simulink model "mrefrobotarm_modified_previous_y_previous_u_previous_ref_prepro"  (R2018b)
settings: Solver=FixedStepAuto  StartTime=0.0  StopTime=10  RelTol=1e-3  AbsTol=1e-6
undefined symbols (not defined in the file or in its folder): cc, options
libraries: neural x594, simulink x1
(part 20 of 22)

== system mrefrobotarm_modified_previous_y_previous_u_previous_ref_prepro/pre_0.001/Layer 3/Delays 1 ==
  "p{3}" : Inport  PortDimensions=30
      mask Display: e = 0.06;c1 = [120 230 180]/255;c2 = ([120 230 180]+0)/(256+128);c3 = ([120 230 180]+128)/(256+128);patch([0 1 1 0],[0 0 1 1],c1);patch([0 1 1 1-e 1-e 0+e],[0 0 1 1-e 0+e 0+e],c2);patch([0 0 1 1-e 0+e 0+e],[0 1 1 1-e 1-e 0+e],c3);plot([0 1 1 0 0],[0 0 1 1 0]);
  mux : Mux  Inputs=1
      mask Display: e = 0.06;c1 = [120 150 230]/255;c2 = ([120 150 230]+0)/383;c3 = ([120 150 230]+128)/383;patch([0 1 1 0],[0 0 1 1],c1);patch([0 1 1 1-e 1-e 0+e],[0 0 1 1-e 0+e 0+e],c2);patch([0 0 1 1-e 0+e 0+e],[0 1 1 1-e 1-e 0+e],c3);plot([0 1 1 0 0],[0 0 1 1 0]);disp('Mux')
  "pd{3,2}" : Outport
      mask Display: e = 0.06;c1 = [120 230 180]/255;c2 = ([120 230 180]+0)/(256+128);c3 = ([120 230 180]+128)/(256+128);patch([0 1 1 0],[0 0 1 1],c1);patch([0 1 1 1-e 1-e 0+e],[0 0 1 1-e 0+e 0+e],c2);patch([0 0 1 1-e 0+e 0+e],[0 1 1 1-e 1-e 0+e],c3);plot([0 1 1 0 0],[0 0 1 1 0]);
  wires:
  "p{3}"/1 -> mux/1
  mux/1 -> "pd{3,2}"/1

== system mrefrobotarm_modified_previous_y_previous_u_previous_ref_prepro/pre_0.001/Layer 3/LW{3,2} ==
  "ad{3,2}" : Inport  PortDimensions=30
      mask Display: e = 0.06;c1 = [120 230 180]/255;c2 = ([120 230 180]+0)/(256+128);c3 = ([120 230 180]+128)/(256+128);patch([0 1 1 0],[0 0 1 1],c1);patch([0 1 1 1-e 1-e 0+e],[0 0 1 1-e 0+e 0+e],c2);patch([0 0 1 1-e 0+e 0+e],[0 1 1 1-e 1-e 0+e],c3);plot([0 1 1 0 0],[0 0 1 1 0]);
  "IW{3,2}(1,:)'" : Constant  Value=[0.436114134671065689641267226761556230485439300537109375;0.4897108664989697768277210343512706458568572998046875;0.265158589575804126692304407697520218789577484130859375;-0.51659794668614644752580034037237055599689483642578125;0.5796996893935404404629707642016001045703887939453125;-0.57276838291900122879241052942234091460704803466796875;0.335826299327664390403924699057824909687042236328125;-0.261032698694444509346368477054056711494922637939453125;0.1045260610150008651064723608214990235865116119384765625;0.49111728847109958895345016571809537708759307861328125;-0.42848603195214407524105126867652870714664459228515625;-0.101925406868263734860846625451813451945781707763671875;-0.175991462046761026893904045209637843072414398193359375;-0.010501595203579773551982867729748249985277652740478515625;0.299745457740388243639273468943429179489612579345703125;-0.1603921728348352282456090733830933459103107452392578125;0.066959779095569327278525406654807738959789276123046875;-0.450890234310093951375364440536941401660442352294921875;-0.51157208381028629329279056037194095551967620849609375;-0.09288836924470354750038580959881073795258998870849609375;0.50675121237872833290794005733914673328399658203125;0.1206441884120259266932606578848208300769329071044921875;0.11866864954212101579411609009184758178889751434326171875;-0.0393519848847962150362178590512485243380069732666015625;-0.242185273598383654647392404513084329664707183837890625;-0.164235090509567693839443336401018314063549041748046875;0.33195926443744749878561606237781234085559844970703125;0.0119212193619771915364946579529714654199779033660888671875;-0.068550038750629205264175425327266566455364227294921875;-0.0692097648270704468576042245331336744129657745361328125]
      mask Display: e = 0.06;c1 = [120 150 230]/255;c2 = ([120 150 230]+0)/383;c3 = ([120 150 230]+128)/383;patch([0 1 1 0],[0 0 1 1],c1);patch([0 1 1 1-e 1-e 0+e],[0 0 1 1-e 0+e 0+e],c2);patch([0 0 1 1-e 0+e 0+e],[0 1 1 1-e 1-e 0+e],c3);plot([0 1 1 0 0],[0 0 1 1 0]);disp('weights');
  Mux : Mux  Inputs=1
      mask Display: e = 0.06;c1 = [120 150 230]/255;c2 = ([120 150 230]+0)/383;c3 = ([120 150 230]+128)/383;patch([0 1 1 0],[0 0 1 1],c1);patch([0 1 1 1-e 1-e 0+e],[0 0 1 1-e 0+e 0+e],c2);patch([0 0 1 1-e 0+e 0+e],[0 1 1 1-e 1-e 0+e],c3);plot([0 1 1 0 0],[0 0 1 1 0]);disp('Mux');
  dotprod1 : neural/Weight Functions/dotprod
  "lz{3,2}" : Outport
      mask Display: e = 0.06;c1 = [120 230 180]/255;c2 = ([120 230 180]+0)/(256+128);c3 = ([120 230 180]+128)/(256+128);patch([0 1 1 0],[0 0 1 1],c1);patch([0 1 1 1-e 1-e 0+e],[0 0 1 1-e 0+e 0+e],c2);patch([0 0 1 1-e 0+e 0+e],[0 1 1 1-e 1-e 0+e],c3);plot([0 1 1 0 0],[0 0 1 1 0]);
  wires:
  "IW{3,2}(1,:)'"/1 -> dotprod1/1
  "ad{3,2}"/1 -> dotprod1/2
  dotprod1/1 -> Mux/1
  Mux/1 -> "lz{3,2}"/1

== system mrefrobotarm_modified_previous_y_previous_u_previous_ref_prepro/pre_0.01/Layer 1/Delays 1 ==
  "p{1}" : Inport  PortDimensions=10
      mask Display: e = 0.06;c1 = [120 230 180]/255;c2 = ([120 230 180]+0)/(256+128);c3 = ([120 230 180]+128)/(256+128);patch([0 1 1 0],[0 0 1 1],c1);patch([0 1 1 1-e 1-e 0+e],[0 0 1 1-e 0+e 0+e],c2);patch([0 0 1 1-e 0+e 0+e],[0 1 1 1-e 1-e 0+e],c3);plot([0 1 1 0 0],[0 0 1 1 0]);
  mux : Mux  Inputs=1
      mask Display: e = 0.06;c1 = [120 150 230]/255;c2 = ([120 150 230]+0)/383;c3 = ([120 150 230]+128)/383;patch([0 1 1 0],[0 0 1 1],c1);patch([0 1 1 1-e 1-e 0+e],[0 0 1 1-e 0+e 0+e],c2);patch([0 0 1 1-e 0+e 0+e],[0 1 1 1-e 1-e 0+e],c3);plot([0 1 1 0 0],[0 0 1 1 0]);disp('Mux')
  "pd{1,1}" : Outport
      mask Display: e = 0.06;c1 = [120 230 180]/255;c2 = ([120 230 180]+0)/(256+128);c3 = ([120 230 180]+128)/(256+128);patch([0 1 1 0],[0 0 1 1],c1);patch([0 1 1 1-e 1-e 0+e],[0 0 1 1-e 0+e 0+e],c2);patch([0 0 1 1-e 0+e 0+e],[0 1 1 1-e 1-e 0+e],c3);plot([0 1 1 0 0],[0 0 1 1 0]);
  wires:
  "p{1}"/1 -> mux/1
  mux/1 -> "pd{1,1}"/1

== system mrefrobotarm_modified_previous_y_previous_u_previous_ref_prepro/pre_0.01/Layer 1/IW{1,1} ==
  "pd{1,1}" : Inport  PortDimensions=10
      mask Display: e = 0.06;c1 = [120 230 180]/255;c2 = ([120 230 180]+0)/(256+128);c3 = ([120 230 180]+128)/(256+128);patch([0 1 1 0],[0 0 1 1],c1);patch([0 1 1 1-e 1-e 0+e],[0 0 1 1-e 0+e 0+e],c2);patch([0 0 1 1-e 0+e 0+e],[0 1 1 1-e 1-e 0+e],c3);plot([0 1 1 0 0],[0 0 1 1 0]);
  "IW{1,1}(1,:)'" : Constant  Value=[-5.85624074115564940967715301667340099811553955078125;3.51680446128212498280163345043547451496124267578125;0.6347381482262941521099719466292299330234527587890625;1.7803816056595789252270378710818476974964141845703125;-1.2333050429232244038502130933920852839946746826171875;-0.1301107597361087775400534383152262307703495025634765625;3.545860369137638468117756929132156074047088623046875;-2.8459252595942228225567305344156920909881591796875;-0.3393944679271430064915193725028075277805328369140625;0.332423639089425126957877409950015135109424591064453125]
      mask Display: e = 0.06;c1 = [120 150 230]/255;c2 = ([120 150 230]+0)/383;c3 = ([120 150 230]+128)/383;patch([0 1 1 0],[0 0 1 1],c1);patch([0 1 1 1-e 1-e 0+e],[0 0 1 1-e 0+e 0+e],c2);patch([0 0 1 1-e 0+e 0+e],[0 1 1 1-e 1-e 0+e],c3);plot([0 1 1 0 0],[0 0 1 1 0]);disp('Weights');
  "IW{1,1}(10,:)'" : Constant  Value=[5.5438114168611445364831524784676730632781982421875;-2.074847987877894706088000020827166736125946044921875;-1.92727949100788986669385849381797015666961669921875;-0.467908740727801586434253522384096868336200714111328125;-2.076676504568512715565020698704756796360015869140625;-0.10576368682021698719442071023877360858023166656494140625;5.00949759583771214721537035075016319751739501953125;-3.03922330836093834705025074072182178497314453125;0.604367742739750468672355054877698421478271484375;-3.819841634701873100965485718916170299053192138671875]
      mask Display: e = 0.06;c1 = [120 150 230]/255;c2 = ([120 150 230]+0)/383;c3 = ([120 150 230]+128)/383;patch([0 1 1 0],[0 0 1 1],c1);patch([0 1 1 1-e 1-e 0+e],[0 0 1 1-e 0+e 0+e],c2);patch([0 0 1 1-e 0+e 0+e],[0 1 1 1-e 1-e 0+e],c3);plot([0 1 1 0 0],[0 0 1 1 0]);disp('Weights');
  "IW{1,1}(11,:)'" : Constant  Value=[1.801450365151530785823297264869324862957000732421875;2.5403773096062547409701437572948634624481201171875;-0.61133654619760935400307744203018955886363983154296875;0.2245239888465724031885173417322221212089061737060546875;-4.25834432503798243629944408894516527652740478515625;-0.456781073421577143989225078257732093334197998046875;1.90877776482296379612080272636376321315765380859375;-0.2448749812280913429329842756487778387963771820068359375;2.974360199360491119335847542970441281795501708984375;0.752977482462759528658580165938474237918853759765625]
      mask Display: e = 0.06;c1 = [120 150 230]/255;c2 = ([120 150 230]+0)/383;c3 = ([120 150 230]+128)/383;patch([0 1 1 0],[0 0 1 1],c1);patch([0 1 1 1-e 1-e 0+e],[0 0 1 1-e 0+e 0+e],c2);patch([0 0 1 1-e 0+e 0+e],[0 1 1 1-e 1-e 0+e],c3);plot([0 1 1 0 0],[0 0 1 1 0]);disp('Weights');
  "IW{1,1}(12,:)'" : Constant  Value=[-5.88547165882157674587915607844479382038116455078125;0.3690016789117473994252804914140142500400543212890625;5.43454272118004677594171880627982318401336669921875;2.021324955409448786980419754399918019771575927734375;3.118231972581463562477210871293209493160247802734375;-4.67881290747909162064388510771095752716064453125;-1.560839517955373789703799047856591641902923583984375;1.316600991380263874219735953374765813350677490234375;-2.9123006538206706039773052907548844814300537109375;-0.36660783874813229754607846189173869788646697998046875]
      mask Display: e = 0.06;c1 = [120 150 230]/255;c2 = ([120 150 230]+0)/383;c3 = ([120 150 230]+128)/383;patch([0 1 1 0],[0 0 1 1],c1);patch([0 1 1 1-e 1-e 0+e],[0 0 1 1-e 0+e 0+e],c2);patch([0 0 1 1-e 0+e 0+e],[0 1 1 1-e 1-e 0+e],c3);plot([0 1 1 0 0],[0 0 1 1 0]);disp('Weights');
  "IW{1,1}(13,:)'" : Constant  Value=[4.4862364253392978952206249232403934001922607421875;-2.21359337096940311795378875103779137134552001953125;-3.6510555857054516337711902451701462268829345703125;-0.59044303803139985831194280763156712055206298828125;4.35225243695406671662340158945880830287933349609375;-0.944076425101286087482321818242780864238739013671875;0.601137947571718456174494349397718906402587890625;-0.9102507336520961889192449234542436897754669189453125;-2.040783866186438810785830355598591268062591552734375;1.14248211452239889496240721200592815876007080078125]
      mask Display: e = 0.06;c1 = [120 150 230]/255;c2 = ([120 150 230]+0)/383;c3 = ([120 150 230]+128)/383;patch([0 1 1 0],[0 0 1 1],c1);patch([0 1 1 1-e 1-e 0+e],[0 0 1 1-e 0+e 0+e],c2);patch([0 0 1 1-e 0+e 0+e],[0 1 1 1-e 1-e 0+e],c3);plot([0 1 1 0 0],[0 0 1 1 0]);disp('Weights');
  "IW{1,1}(14,:)'" : Constant  Value=[2.96005758962551634994042615289799869060516357421875;-2.628426232952859376013066139421425759792327880859375;0.9426964090625158387837245754781179130077362060546875;-2.009528625793982836711393247242085635662078857421875;4.98013932269017356446738631348125636577606201171875;-2.84339358174093081998989873682148754596710205078125;-1.499753220486744975659121337230317294597625732421875;0.61186224711551628896444299243739806115627288818359375;-0.91867019710147157507407200682791881263256072998046875;-1.1056470699375766653105301884352229535579681396484375]
      mask Display: e = 0.06;c1 = [120 150 230]/255;c2 = ([120 150 230]+0)/383;c3 = ([120 150 230]+128)/383;patch([0 1 1 0],[0 0 1 1],c1);patch([0 1 1 1-e 1-e 0+e],[0 0 1 1-e 0+e 0+e],c2);patch([0 0 1 1-e 0+e 0+e],[0 1 1 1-e 1-e 0+e],c3);plot([0 1 1 0 0],[0 0 1 1 0]);disp('Weights');
  "IW{1,1}(15,:)'" : Constant  Value=[1.3405973719274850708416124689392745494842529296875;-0.94740730540068518461538360497797839343547821044921875;-0.8051968085434351163343080770573578774929046630859375;0.8401875525177968651036053415737114846706390380859375;-2.38333203591385522912560190889053046703338623046875;2.247255001731979451307097406242974102497100830078125;-2.1907243293222418145660412847064435482025146484375;1.393962444028848945976051254547201097011566162109375;-2.9782811404097788710032546077854931354522705078125;-3.071191113830036290011094024521298706531524658203125]
      mask Display: e = 0.06;c1 = [120 150 230]/255;c2 = ([120 150 230]+0)/383;c3 = ([120 150 230]+128)/383;patch([0 1 1 0],[0 0 1 1],c1);patch([0 1 1 1-e 1-e 0+e],[0 0 1 1-e 0+e 0+e],c2);patch([0 0 1 1-e 0+e 0+e],[0 1 1 1-e 1-e 0+e],c3);plot([0 1 1 0 0],[0 0 1 1 0]);disp('Weights');
  "IW{1,1}(16,:)'" : Constant  Value=[5.24956005510203294051052580471150577068328857421875;-3.123270889222998558665267410106025636196136474609375;-2.899628478866194125629363043117336928844451904296875;1.2721033387022446792258278946974314749240875244140625;-6.7373528318352189359075055108405649662017822265625;4.95546573290953151769144824356772005558013916015625;0.53229393194607588224442906721378676593303680419921875;1.3107157379762164328695916992728598415851593017578125;-6.4141498126504306043216274701990187168121337890625;-1.688800676216443807931000264943577349185943603515625]
      mask Display: e = 0.06;c1 = [120 150 230]/255;c2 = ([120 150 230]+0)/383;c3 = ([120 150 230]+128)/383;patch([0 1 1 0],[0 0 1 1],c1);patch([0 1 1 1-e 1-e 0+e],[0 0 1 1-e 0+e 0+e],c2);patch([0 0 1 1-e 0+e 0+e],[0 1 1 1-e 1-e 0+e],c3);plot([0 1 1 0 0],[0 0 1 1 0]);disp('Weights');
  "IW{1,1}(17,:)'" : Constant  Value=[0.402854375334637915262447904751752503216266632080078125;-1.9260767289406282021246852309559471905231475830078125;0.78951047299180476812807683018036186695098876953125;0.68164611125391871837564394809305667877197265625;-0.634424106110297092442351640784181654453277587890625;0.1365768899834514382707340018896502442657947540283203125;1.9467877645893822968758968272595666348934173583984375;-0.913545588347322468081301849451847374439239501953125;1.6488021045101197703530715443775989115238189697265625;-0.22812449883821361851232722983695566654205322265625]
      mask Display: e = 0.06;c1 = [120 150 230]/255;c2 = ([120 150 230]+0)/383;c3 = ([120 150 230]+128)/383;patch([0 1 1 0],[0 0 1 1],c1);patch([0 1 1 1-e 1-e 0+e],[0 0 1 1-e 0+e 0+e],c2);patch([0 0 1 1-e 0+e 0+e],[0 1 1 1-e 1-e 0+e],c3);plot([0 1 1 0 0],[0 0 1 1 0]);disp('Weights');
  "IW{1,1}(18,:)'" : Constant  Value=[-3.926344015276355126076168744475580751895904541015625;2.64736178851262682343303822563029825687408447265625;1.4944123035889393946717973449267446994781494140625;-1.548625935119756658053802311769686639308929443359375;2.158669751416033566471242011175490915775299072265625;-0.3860689796058196510131210743566043674945831298828125;-1.255149649516599463794364055502228438854217529296875;0.5499562614605004728929316115682013332843780517578125;1.4076190893442135365631884269532747566699981689453125;-1.68961743441577372237816234701313078403472900390625]
      mask Display: e = 0.06;c1 = [120 150 230]/255;c2 = ([120 150 230]+0)/383;c3 = ([120 150 230]+128)/383;patch([0 1 1 0],[0 0 1 1],c1);patch([0 1 1 1-e 1-e 0+e],[0 0 1 1-e 0+e 0+e],c2);patch([0 0 1 1-e 0+e 0+e],[0 1 1 1-e 1-e 0+e],c3);plot([0 1 1 0 0],[0 0 1 1 0]);disp('Weights');
  "IW{1,1}(19,:)'" : Constant  Value=[-8.6575548675962945566197959124110639095306396484375;4.10379744179784466950877686031162738800048828125;-0.327724649637724685380391065336880274116992950439453125;3.97567807798125461005156466853804886341094970703125;3.70194788223165627272237543365918099880218505859375;-1.2007687177355277352575058102956973016262054443359375;-2.094451910380683568035919961403124034404754638671875;0.6931746778662428720707566753844730556011199951171875;0.390829399024751278357570072330418042838573455810546875;3.424383189735958676891414143028669059276580810546875]
      mask Display: e = 0.06;c1 = [120 150 230]/255;c2 = ([120 150 230]+0)/383;c3 = ([120 150 230]+128)/383;patch([0 1 1 0],[0 0 1 1],c1);patch([0 1 1 1-e 1-e 0+e],[0 0 1 1-e 0+e 0+e],c2);patch([0 0 1 1-e 0+e 0+e],[0 1 1 1-e 1-e 0+e],c3);plot([0 1 1 0 0],[0 0 1 1 0]);disp('Weights');
  "IW{1,1}(2,:)'" : Constant  Value=[2.6125118629305763562342690420337021350860595703125;-1.37514288325557654246722449897788465023040771484375;-1.401681826106581763013991803745739161968231201171875;0.83219132133275397489313718324410729110240936279296875;-1.953893972122157318693780325702391564846038818359375;0.69612144520550833792782441378221847116947174072265625;1.7696692580941599803878716556937433779239654541015625;-1.5785633815546535885232515283860266208648681640625;-3.442944793421773841402000471134670078754425048828125;0.68140069773722711232721849228255450725555419921875]
      mask Display: e = 0.06;c1 = [120 150 230]/255;c2 = ([120 150 230]+0)/383;c3 = ([120 150 230]+128)/383;patch([0 1 1 0],[0 0 1 1],c1);patch([0 1 1 1-e 1-e 0+e],[0 0 1 1-e 0+e 0+e],c2);patch([0 0 1 1-e 0+e 0+e],[0 1 1 1-e 1-e 0+e],c3);plot([0 1 1 0 0],[0 0 1 1 0]);disp('Weights');
  "IW{1,1}(20,:)'" : Constant  Value=[-5.82456522810500754161466829827986657619476318359375;4.77771073300586035514925242750905454158782958984375;2.22666821103919065905074603506363928318023681640625;-2.07154279514932770922541749314405024051666259765625;1.984621844522302058777540878509171307086944580078125;0.81260359941105109182757360031246207654476165771484375;-1.7979220800818911385476894793100655078887939453125;-0.19148413309093204048849656828679144382476806640625;3.266091133828860737509103273623622953891754150390625;-0.423175203307374736549917315642233006656169891357421875]
      mask Display: e = 0.06;c1 = [120 150 230]/255;c2 = ([120 150 230]+0)/383;c3 = ([120 150 230]+128)/383;patch([0 1 1 0],[0 0 1 1],c1);patch([0 1 1 1-e 1-e 0+e],[0 0 1 1-e 0+e 0+e],c2);patch([0 0 1 1-e 0+e 0+e],[0 1 1 1-e 1-e 0+e],c3);plot([0 1 1 0 0],[0 0 1 1 0]);disp('Weights');
  "IW{1,1}(21,:)'" : Constant  Value=[-2.6788162832066291230148635804653167724609375;1.531265910973661714677973577636294066905975341796875;-1.2272697973190014320010732262744568288326263427734375;0.2462738275440067570176694289330043829977512359619140625;3.7563299795286670956784291774965822696685791015625;-2.676750026289990369576798912021331489086151123046875;2.749977990810542838318042413447983562946319580078125;-2.43343537079067306905244549852795898914337158203125;-3.120985268643997390114463996724225580692291259765625;1.3113749338071869487976073287427425384521484375]
      mask Display: e = 0.06;c1 = [120 150 230]/255;c2 = ([120 150 230]+0)/383;c3 = ([120 150 230]+128)/383;patch([0 1 1 0],[0 0 1 1],c1);patch([0 1 1 1-e 1-e 0+e],[0 0 1 1-e 0+e 0+e],c2);patch([0 0 1 1-e 0+e 0+e],[0 1 1 1-e 1-e 0+e],c3);plot([0 1 1 0 0],[0 0 1 1 0]);disp('Weights');
  "IW{1,1}(22,:)'" : Constant  Value=[-2.331678787855488987901253494783304631710052490234375;1.9175273555104686007410919046378694474697113037109375;2.785754327334096114299200053210370242595672607421875;1.220232959880296785826203631586395204067230224609375;3.930124642441815918658676309860311448574066162109375;-0.9763831564017639852437469016877003014087677001953125;-0.5288300752090524525783621356822550296783447265625;-0.53467152456522060166577148265787400305271148681640625;3.027168159407801706350937820388935506343841552734375;-2.546789484386377200308970714104361832141876220703125]
      mask Display: e = 0.06;c1 = [120 150 230]/255;c2 = ([120 150 230]+0)/383;c3 = ([120 150 230]+128)/383;patch([0 1 1 0],[0 0 1 1],c1);patch([0 1 1 1-e 1-e 0+e],[0 0 1 1-e 0+e 0+e],c2);patch([0 0 1 1-e 0+e 0+e],[0 1 1 1-e 1-e 0+e],c3);plot([0 1 1 0 0],[0 0 1 1 0]);disp('Weights');
  "IW{1,1}(23,:)'" : Constant  Value=[-3.297749992552132969336753376410342752933502197265625;0.95345391607309759596233789125108160078525543212890625;1.3085273842947042766127196955494582653045654296875;-2.09606923060831373817336498177610337734222412109375;0.6649085374571017670319861281313933432102203369140625;-2.605191632574497706542615560465492308139801025390625;-0.2086664202659928302185932125212275423109531402587890625;0.29301975068497665422029285764438100159168243408203125;0.0533424003255774381582199339391081593930721282958984375;-0.9746507344559234287117988060344941914081573486328125]
      mask Display: e = 0.06;c1 = [120 150 230]/255;c2 = ([120 150 230]+0)/383;c3 = ([120 150 230]+128)/383;patch([0 1 1 0],[0 0 1 1],c1);patch([0 1 1 1-e 1-e 0+e],[0 0 1 1-e 0+e 0+e],c2);patch([0 0 1 1-e 0+e 0+e],[0 1 1 1-e 1-e 0+e],c3);plot([0 1 1 0 0],[0 0 1 1 0]);disp('Weights');
  "IW{1,1}(24,:)'" : Constant  Value=[5.26403541711713796047433788771741092205047607421875;-4.350305274247940445775384432636201381683349609375;-2.446240935645905612005890361615456640720367431640625;0.281055804546570364710333933544461615383625030517578125;1.50024635213031043434739331132732331752777099609375;-4.03994831318534775022044414072297513484954833984375;-1.835789247584131533841400596429593861103057861328125;1.1544983756443236710964583835448138415813446044921875;1.348684999744826473744296890799887478351593017578125;-2.47782798748131316557419268065132200717926025390625]
      mask Display: e = 0.06;c1 = [120 150 230]/255;c2 = ([120 150 230]+0)/383;c3 = ([120 150 230]+128)/383;patch([0 1 1 0],[0 0 1 1],c1);patch([0 1 1 1-e 1-e 0+e],[0 0 1 1-e 0+e 0+e],c2);patch([0 0 1 1-e 0+e 0+e],[0 1 1 1-e 1-e 0+e],c3);plot([0 1 1 0 0],[0 0 1 1 0]);disp('Weights');
  "IW{1,1}(25,:)'" : Constant  Value=[-3.7163175636467347118241377756930887699127197265625;0.52039148612197172472093598116771318018436431884765625;0.62464525370229118106379928576643578708171844482421875;1.1292601515886386831510890260688029229640960693359375;4.03204641347660075467729257070459425449371337890625;-3.35339086600971025831086080870591104030609130859375;-0.67736203672771699846322235316620208323001861572265625;1.1033568521567953535367223594221286475658416748046875;2.1720579810827533862038762890733778476715087890625;0.294348933198287754375854774480103515088558197021484375]
      mask Display: e = 0.06;c1 = [120 150 230]/255;c2 = ([120 150 230]+0)/383;c3 = ([120 150 230]+128)/383;patch([0 1 1 0],[0 0 1 1],c1);patch([0 1 1 1-e 1-e 0+e],[0 0 1 1-e 0+e 0+e],c2);patch([0 0 1 1-e 0+e 0+e],[0 1 1 1-e 1-e 0+e],c3);plot([0 1 1 0 0],[0 0 1 1 0]);disp('Weights');
  "IW{1,1}(26,:)'" : Constant  Value=[7.68110421554345013106512851663865149021148681640625;-5.5806375133580292668966649216599762439727783203125;0.6474186917384816553067139466293156147003173828125;-0.25813591302558880347106651242938823997974395751953125;-7.25354088639611660482842125929892063140869140625;2.34772948867883091139674434089101850986480712890625;2.008143539473588479182808441692031919956207275390625;0.328548453086462022287861373115447349846363067626953125;0.66391334420801617621776813393807969987392425537109375;-1.7681702103446050866608629803522489964962005615234375]
      mask Display: e = 0.06;c1 = [120 150 230]/255;c2 = ([120 150 230]+0)/383;c3 = ([120 150 230]+128)/383;patch([0 1 1 0],[0 0 1 1],c1);patch([0 1 1 1-e 1-e 0+e],[0 0 1 1-e 0+e 0+e],c2);patch([0 0 1 1-e 0+e 0+e],[0 1 1 1-e 1-e 0+e],c3);plot([0 1 1 0 0],[0 0 1 1 0]);disp('Weights');
  "IW{1,1}(27,:)'" : Constant  Value=[-3.88890360968008419462194069637916982173919677734375;1.807719452135531756908903844305314123630523681640625;1.8443906482025564930182781608891673386096954345703125;0.05960729976508481742225598054574220441281795501708984375;6.41662600072029309927756912657059729099273681640625;-4.731342225276449653392774052917957305908203125;-1.9683220855801606408164161621243692934513092041015625;-0.155691989537033170787339031448937021195888519287109375;1.5052831323353388359720383959938772022724151611328125;3.0499443373096735143690239056013524532318115234375]
      mask Display: e = 0.06;c1 = [120 150 230]/255;c2 = ([120 150 230]+0)/383;c3 = ([120 150 230]+128)/383;patch([0 1 1 0],[0 0 1 1],c1);patch([0 1 1 1-e 1-e 0+e],[0 0 1 1-e 0+e 0+e],c2);patch([0 0 1 1-e 0+e 0+e],[0 1 1 1-e 1-e 0+e],c3);plot([0 1 1 0 0],[0 0 1 1 0]);disp('Weights');
  "IW{1,1}(28,:)'" : Constant  Value=[-2.08873314887912808757164384587667882442474365234375;-2.177558277080478443821220935205928981304168701171875;1.85911414065590374633529791026376187801361083984375;0.7786322163372434435046898215659894049167633056640625;-2.878435651152690955001389738754369318485260009765625;0.85485495305713066205299810462747700512409210205078125;-0.544214717952030024861187484930269420146942138671875;1.2201975643732592136103676239144988358020782470703125;1.9343350066125617470191855318262241780757904052734375;-0.1590528401144102321751461204257793724536895751953125]
      mask Display: e = 0.06;c1 = [120 150 230]/255;c2 = ([120 150 230]+0)/383;c3 = ([120 150 230]+128)/383;patch([0 1 1 0],[0 0 1 1],c1);patch([0 1 1 1-e 1-e 0+e],[0 0 1 1-e 0+e 0+e],c2);patch([0 0 1 1-e 0+e 0+e],[0 1 1 1-e 1-e 0+e],c3);plot([0 1 1 0 0],[0 0 1 1 0]);disp('Weights');
  "IW{1,1}(29,:)'" : Constant  Value=[-3.3140155268266173749225345090962946414947509765625;2.22866180250222978287411024211905896663665771484375;-0.20167459266773357651203468776657246053218841552734375;-0.1575369015674890904588067996883182786405086517333984375;-3.381821830384472260533357257372699677944183349609375;1.2952284826152082874983761939802207052707672119140625;-1.1796565663488285391480303587741218507289886474609375;3.439748069590938595041507142013870179653167724609375;-3.675285077898163610399251410854049026966094970703125;-2.262756383297438222967912224703468382358551025390625]
      mask Display: e = 0.06;c1 = [120 150 230]/255;c2 = ([120 150 230]+0)/383;c3 = ([120 150 230]+128)/383;patch([0 1 1 0],[0 0 1 1],c1);patch([0 1 1 1-e 1-e 0+e],[0 0 1 1-e 0+e 0+e],c2);patch([0 0 1 1-e 0+e 0+e],[0 1 1 1-e 1-e 0+e],c3);plot([0 1 1 0 0],[0 0 1 1 0]);disp('Weights');
  "IW{1,1}(3,:)'" : Constant  Value=[-0.56675888134729401901523715423536486923694610595703125;-0.34119466903833195470241435032221488654613494873046875;-0.39663512936999711921970401817816309630870819091796875;0.478829072563840885123909174581058323383331298828125;-3.366711754555829383406262422795407474040985107421875;3.2339992215156403432274601073004305362701416015625;-1.1517120277756067725505317866918630897998809814453125;1.4794355264062897248322769883088767528533935546875;-4.24056030156204588621449147467501461505889892578125;1.210775540611519485167946186265908181667327880859375]
      mask Display: e = 0.06;c1 = [120 150 230]/255;c2 = ([120 150 230]+0)/383;c3 = ([120 150 230]+128)/383;patch([0 1 1 0],[0 0 1 1],c1);patch([0 1 1 1-e 1-e 0+e],[0 0 1 1-e 0+e 0+e],c2);patch([0 0 1 1-e 0+e 0+e],[0 1 1 1-e 1-e 0+e],c3);plot([0 1 1 0 0],[0 0 1 1 0]);disp('Weights');
  "IW{1,1}(30,:)'" : Constant  Value=[-1.2533905500174207237051859920029528439044952392578125;-1.0861989916824443813681000392534770071506500244140625;1.396198612017170770371876642457209527492523193359375;2.860837090867893284240608409163542091846466064453125;-2.472957936277264234803396902862004935741424560546875;1.3823525587225502508914587451727129518985748291015625;-1.142285625577001528796472484827972948551177978515625;0.9551498948774297392816379215219058096408843994140625;1.1108403503011061719263352642883546650409698486328125;2.648168806111362183486335197812877595424652099609375]
      mask Display: e = 0.06;c1 = [120 150 230]/255;c2 = ([120 150 230]+0)/383;c3 = ([120 150 230]+128)/383;patch([0 1 1 0],[0 0 1 1],c1);patch([0 1 1 1-e 1-e 0+e],[0 0 1 1-e 0+e 0+e],c2);patch([0 0 1 1-e 0+e 0+e],[0 1 1 1-e 1-e 0+e],c3);plot([0 1 1 0 0],[0 0 1 1 0]);disp('Weights');
  "IW{1,1}(4,:)'" : Constant  Value=[-6.5853133771012029029634504695422947406768798828125;2.76263961904087285148534647305496037006378173828125;0.30869851091883881988309212829335592687129974365234375;0.4193313033892469565699911981937475502490997314453125;2.316828555632335362446383442147634923458099365234375;-1.1864510017739362535138525345246307551860809326171875;-0.485024537478817074909187567754997871816158294677734375;0.461871944816222346208434146319632418453693389892578125;0.433714380881770000808472786957281641662120819091796875;-3.204995011492357104287975744227878749370574951171875]
      mask Display: e = 0.06;c1 = [120 150 230]/255;c2 = ([120 150 230]+0)/383;c3 = ([120 150 230]+128)/383;patch([0 1 1 0],[0 0 1 1],c1);patch([0 1 1 1-e 1-e 0+e],[0 0 1 1-e 0+e 0+e],c2);patch([0 0 1 1-e 0+e 0+e],[0 1 1 1-e 1-e 0+e],c3);plot([0 1 1 0 0],[0 0 1 1 0]);disp('Weights');
  "IW{1,1}(5,:)'" : Constant  Value=[5.73852534707076689102223099325783550739288330078125;0.05805293153485781287859168742215842939913272857666015625;-3.04412521841268546296532804262824356555938720703125;-0.503981225017013922951036875019781291484832763671875;-2.549002892817883836329428959288634359836578369140625;3.2228411095297833099948547896929085254669189453125;0.97345814077867931501941711758263409137725830078125;-3.787924656487893226852747829980216920375823974609375;-0.60928514859972071615601407756912522017955780029296875;2.183424672023919210772646692930720746517181396484375]
      mask Display: e = 0.06;c1 = [120 150 230]/255;c2 = ([120 150 230]+0)/383;c3 = ([120 150 230]+128)/383;patch([0 1 1 0],[0 0 1 1],c1);patch([0 1 1 1-e 1-e 0+e],[0 0 1 1-e 0+e 0+e],c2);patch([0 0 1 1-e 0+e 0+e],[0 1 1 1-e 1-e 0+e],c3);plot([0 1 1 0 0],[0 0 1 1 0]);disp('Weights');
  "IW{1,1}(6,:)'" : Constant  Value=[-2.217512967826573255791799965663813054561614990234375;-0.58904066927541298692716509322053752839565277099609375;-2.49048429040009455803783566807396709918975830078125;-2.4578114385713103473563023726455867290496826171875;3.312526560791344110157297109253704547882080078125;1.2083392816733609098633905887254513800144195556640625;1.602648226646122164851249181083403527736663818359375;-0.067456206185177391976282024188549257814884185791015625;-1.8774466036302548399561374026234261691570281982421875;0.94688616102039180333349577267654240131378173828125]
      mask Display: e = 0.06;c1 = [120 150 230]/255;c2 = ([120 150 230]+0)/383;c3 = ([120 150 230]+128)/383;patch([0 1 1 0],[0 0 1 1],c1);patch([0 1 1 1-e 1-e 0+e],[0 0 1 1-e 0+e 0+e],c2);patch([0 0 1 1-e 0+e 0+e],[0 1 1 1-e 1-e 0+e],c3);plot([0 1 1 0 0],[0 0 1 1 0]);disp('Weights');
  "IW{1,1}(7,:)'" : Constant  Value=[-1.089049180437282604572146738064475357532501220703125;1.255433125095382518310316299903206527233123779296875;2.4781431225701648912718155770562589168548583984375;-1.0194681182791718310198803010280244052410125732421875;2.630481406433080149298575634020380675792694091796875;0.320844367893274695635597026921459473669528961181640625;2.25318642433378268918886533356271684169769287109375;0.475399692536651985452778035323717631399631500244140625;-2.68939142291155430797289227484725415706634521484375;-2.788639261698481863760434862342663109302520751953125]
      mask Display: e = 0.06;c1 = [120 150 230]/255;c2 = ([120 150 230]+0)/383;c3 = ([120 150 230]+128)/383;patch([0 1 1 0],[0 0 1 1],c1);patch([0 1 1 1-e 1-e 0+e],[0 0 1 1-e 0+e 0+e],c2);patch([0 0 1 1-e 0+e 0+e],[0 1 1 1-e 1-e 0+e],c3);plot([0 1 1 0 0],[0 0 1 1 0]);disp('Weights');
  "IW{1,1}(8,:)'" : Constant  Value=[2.392262476918522562385760465986095368862152099609375;0.177484958916592716615667768564890138804912567138671875;-1.7835335264594878168509239912964403629302978515625;0.0140831422173770814953996932672453112900257110595703125;2.43462897912698306157608385547064244747161865234375;0.29665149320045369751852604167652316391468048095703125;0.399042029318930235870510614404338411986827850341796875;-3.16678935948543571754498771042563021183013916015625;2.0553687128479456447394113638438284397125244140625;0.1463976569483515788316907446642289869487285614013671875]
      mask Display: e = 0.06;c1 = [120 150 230]/255;c2 = ([120 150 230]+0)/383;c3 = ([120 150 230]+128)/383;patch([0 1 1 0],[0 0 1 1],c1);patch([0 1 1 1-e 1-e 0+e],[0 0 1 1-e 0+e 0+e],c2);patch([0 0 1 1-e 0+e 0+e],[0 1 1 1-e 1-e 0+e],c3);plot([0 1 1 0 0],[0 0 1 1 0]);disp('Weights');
  "IW{1,1}(9,:)'" : Constant  Value=[5.0927416790097854715213543386198580265045166015625;-0.50360252949831874058617131595383398234844207763671875;-1.906654036515735839429908082820475101470947265625;-1.400523239361530780655584749183617532253265380859375;2.73113887691750534258972038514912128448486328125;-5.388534158780228011664803489111363887786865234375;1.99641404741776540276987361721694469451904296875;0.1001455352311608759663386081228964030742645263671875;-0.427650648383573306343663489315076731145381927490234375;-1.7623339402115936191961509393877349793910980224609375]
      mask Display: e = 0.06;c1 = [120 150 230]/255;c2 = ([120 150 230]+0)/383;c3 = ([120 150 230]+128)/383;patch([0 1 1 0],[0 0 1 1],c1);patch([0 1 1 1-e 1-e 0+e],[0 0 1 1-e 0+e 0+e],c2);patch([0 0 1 1-e 0+e 0+e],[0 1 1 1-e 1-e 0+e],c3);plot([0 1 1 0 0],[0 0 1 1 0]);disp('Weights');
  Mux : Mux  Inputs=30
      mask Display: e = 0.06;c1 = [120 150 230]/255;c2 = ([120 150 230]+0)/383;c3 = ([120 150 230]+128)/383;patch([0 1 1 0],[0 0 1 1],c1);patch([0 1 1 1-e 1-e 0+e],[0 0 1 1-e 0+e 0+e],c2);patch([0 0 1 1-e 0+e 0+e],[0 1 1 1-e 1-e 0+e],c3);plot([0 1 1 0 0],[0 0 1 1 0]);disp('Mux');
  dotprod{1..30} (30 alike) : neural/Weight Functions/dotprod
  "iz{1,1}" : Outport
      mask Display: e = 0.06;c1 = [120 230 180]/255;c2 = ([120 230 180]+0)/(256+128);c3 = ([120 230 180]+128)/(256+128);patch([0 1 1 0],[0 0 1 1],c1);patch([0 1 1 1-e 1-e 0+e],[0 0 1 1-e 0+e 0+e],c2);patch([0 0 1 1-e 0+e 0+e],[0 1 1 1-e 1-e 0+e],c3);plot([0 1 1 0 0],[0 0 1 1 0]);
  wires:
  "IW{1,1}(1,:)'"/1 -> dotprod1/1
  "pd{1,1}"/1 -> dotprod1/2, dotprod2/2, dotprod3/2, dotprod4/2, dotprod5/2, dotprod6/2, dotprod7/2, dotprod8/2, dotprod9/2, dotprod10/2, dotprod11/2, dotprod12/2, dotprod13/2, dotprod14/2, dotprod15/2, dotprod16/2, dotprod17/2, dotprod18/2, dotprod19/2, dotprod20/2, dotprod21/2, dotprod22/2, dotprod23/2, dotprod24/2, dotprod25/2, dotprod26/2, dotprod27/2, dotprod28/2, dotprod29/2, dotprod30/2
  dotprod1/1 -> Mux/1
  "IW{1,1}(2,:)'"/1 -> dotprod2/1
  dotprod2/1 -> Mux/2
  "IW{1,1}(3,:)'"/1 -> dotprod3/1
  dotprod3/1 -> Mux/3
  "IW{1,1}(4,:)'"/1 -> dotprod4/1
  dotprod4/1 -> Mux/4
  "IW{1,1}(5,:)'"/1 -> dotprod5/1
  dotprod5/1 -> Mux/5
  "IW{1,1}(6,:)'"/1 -> dotprod6/1
  dotprod6/1 -> Mux/6
  "IW{1,1}(7,:)'"/1 -> dotprod7/1
  dotprod7/1 -> Mux/7
  "IW{1,1}(8,:)'"/1 -> dotprod8/1
  dotprod8/1 -> Mux/8
  "IW{1,1}(9,:)'"/1 -> dotprod9/1
  dotprod9/1 -> Mux/9
  "IW{1,1}(10,:)'"/1 -> dotprod10/1
  dotprod10/1 -> Mux/10
  "IW{1,1}(11,:)'"/1 -> dotprod11/1
  dotprod11/1 -> Mux/11
  "IW{1,1}(12,:)'"/1 -> dotprod12/1
  dotprod12/1 -> Mux/12
  "IW{1,1}(13,:)'"/1 -> dotprod13/1
  dotprod13/1 -> Mux/13
  "IW{1,1}(14,:)'"/1 -> dotprod14/1
  dotprod14/1 -> Mux/14
  "IW{1,1}(15,:)'"/1 -> dotprod15/1
  dotprod15/1 -> Mux/15
  "IW{1,1}(16,:)'"/1 -> dotprod16/1
  dotprod16/1 -> Mux/16
  "IW{1,1}(17,:)'"/1 -> dotprod17/1
  dotprod17/1 -> Mux/17
  "IW{1,1}(18,:)'"/1 -> dotprod18/1
  dotprod18/1 -> Mux/18
  "IW{1,1}(19,:)'"/1 -> dotprod19/1
  dotprod19/1 -> Mux/19
  "IW{1,1}(20,:)'"/1 -> dotprod20/1
  dotprod20/1 -> Mux/20
  "IW{1,1}(21,:)'"/1 -> dotprod21/1
  dotprod21/1 -> Mux/21
  "IW{1,1}(22,:)'"/1 -> dotprod22/1
  dotprod22/1 -> Mux/22
  "IW{1,1}(23,:)'"/1 -> dotprod23/1
  dotprod23/1 -> Mux/23
  "IW{1,1}(24,:)'"/1 -> dotprod24/1
  dotprod24/1 -> Mux/24
  "IW{1,1}(25,:)'"/1 -> dotprod25/1
  dotprod25/1 -> Mux/25
  "IW{1,1}(26,:)'"/1 -> dotprod26/1
  dotprod26/1 -> Mux/26
  "IW{1,1}(27,:)'"/1 -> dotprod27/1
  dotprod27/1 -> Mux/27
  "IW{1,1}(28,:)'"/1 -> dotprod28/1
  dotprod28/1 -> Mux/28
  "IW{1,1}(29,:)'"/1 -> dotprod29/1
  dotprod29/1 -> Mux/29
  "IW{1,1}(30,:)'"/1 -> dotprod30/1
  dotprod30/1 -> Mux/30
  Mux/1 -> "iz{1,1}"/1

== system mrefrobotarm_modified_previous_y_previous_u_previous_ref_prepro/pre_0.01/Layer 2/Delays 1 ==
  "p{2}" : Inport  PortDimensions=30
      mask Display: e = 0.06;c1 = [120 230 180]/255;c2 = ([120 230 180]+0)/(256+128);c3 = ([120 230 180]+128)/(256+128);patch([0 1 1 0],[0 0 1 1],c1);patch([0 1 1 1-e 1-e 0+e],[0 0 1 1-e 0+e 0+e],c2);patch([0 0 1 1-e 0+e 0+e],[0 1 1 1-e 1-e 0+e],c3);plot([0 1 1 0 0],[0 0 1 1 0]);
  mux : Mux  Inputs=1
      mask Display: e = 0.06;c1 = [120 150 230]/255;c2 = ([120 150 230]+0)/383;c3 = ([120 150 230]+128)/383;patch([0 1 1 0],[0 0 1 1],c1);patch([0 1 1 1-e 1-e 0+e],[0 0 1 1-e 0+e 0+e],c2);patch([0 0 1 1-e 0+e 0+e],[0 1 1 1-e 1-e 0+e],c3);plot([0 1 1 0 0],[0 0 1 1 0]);disp('Mux')
  "pd{2,1}" : Outport
      mask Display: e = 0.06;c1 = [120 230 180]/255;c2 = ([120 230 180]+0)/(256+128);c3 = ([120 230 180]+128)/(256+128);patch([0 1 1 0],[0 0 1 1],c1);patch([0 1 1 1-e 1-e 0+e],[0 0 1 1-e 0+e 0+e],c2);patch([0 0 1 1-e 0+e 0+e],[0 1 1 1-e 1-e 0+e],c3);plot([0 1 1 0 0],[0 0 1 1 0]);
  wires:
  "p{2}"/1 -> mux/1
  mux/1 -> "pd{2,1}"/1
